simulink model "Simple_Model_Packaging_7_1"  (R2022b)
settings: Solver=VariableStepAuto  StartTime=0.0  StopTime=0.01  RelTol=1e-3
InitFcn:
  | Parameter_Initialize_7
undefined symbols (not defined in the file or in its folder): gcbh, magnitude, model, rcfiltgaincompat
libraries: simulink x2, commdigbbndfm2 x1, commdigbbndam3 x1, commfilt2 x1
settings Model: Creator=89778  LastModifiedBy=z0y

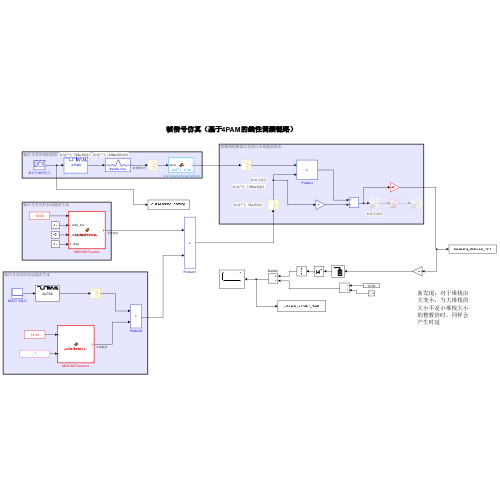
[thumbnail: Simulink's stored preview of the top-level diagram]
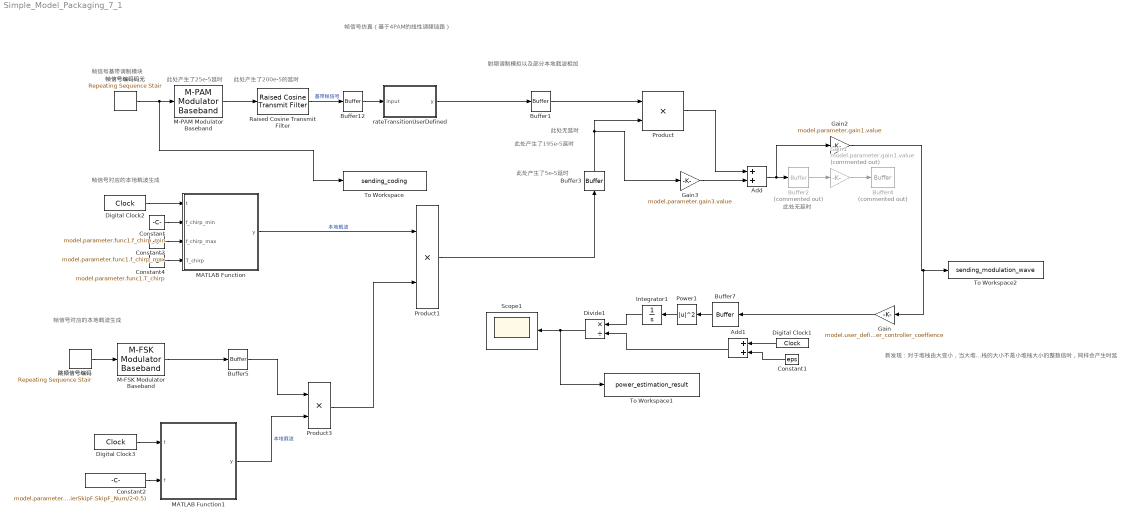
== system Simple_Model_Packaging_7_1 ==
  note: 帧信号仿真（基于4PAM的线性调频链路）
  note: 新发现：对于堆栈由大变小，当大堆栈的大小不是小堆栈大小的整数倍时，同样会产生时延
  note: 此处无延时
  note: 此处产生了25e-5延时
  note: 帧信号基带调制模块
  note: 此处产生了200e-5的延时
  note: 帧信号对应的本地载波生成
  note: 此处产生了195e-5延时
  note: 射频调制模拟以及部分本地载波相加
  note: 此处产生了5e-5延时
  note: 此处无延时
  note: 帧信号对应的本地载波生成
  Add : Sum
  Add1 : Sum
  Buffer1 : Buffer  N=model.parameter.Buffer1.Output_buffer_size  OutputFrames=off
  Buffer12 : Buffer  N=model.parameter.Buffer12.Output_buffer_size  OutputFrames=off
  Buffer2 : Buffer  Commented=on  N=model.parameter.Buffer2.Output_buffer_size  OutputFrames=off
  Buffer3 : Buffer  N=model.parameter.Buffer3.Output_buffer_size  OutputFrames=off
  Buffer4 : Buffer  Commented=on  N=model.parameter.Buffer4.Output_buffer_size  OutputFrames=off
  Buffer5 : Buffer  N=1  OutputFrames=off
  Buffer7 : Buffer  N=1  OutputFrames=off
  Constant : Constant  Value=model.parameter.func1.f_chirp_min
  Constant1 : Constant  Value=eps  SampleTime=model.parameter.channel_estimate_fs
  Constant2 : Constant  Value=model.parameter.CarrierSkipF.SkipF_distance*(model.parameter.CarrierSkipF.SkipF_Num/2-0.5)
  Constant3 : Constant  Value=model.parameter.func1.f_chirp_max
  Constant4 : Constant  Value=model.parameter.func1.T_chirp
  Digital Clock1 : DigitalClock  SampleTime=model.parameter.channel_estimate_fs
  Digital Clock2 : DigitalClock  SampleTime=model.parameter.Digital_Clock2.CarrierTs
  Digital Clock3 : DigitalClock  SampleTime=model.parameter.Digital_Clock2.CarrierTs
  Divide1 : Product  Inputs=*/
  Gain : Gain  Gain=model.user_defined.TR.Sig_power_controller_coeffience
  Gain1 : Gain  Commented=on  Gain=model.parameter.gain1.value
  Gain2 : Gain  Gain=model.parameter.gain1.value
  Gain3 : Gain  Gain=model.parameter.gain3.value
  Integrator1 : Integrator
  M-FSK Modulator Baseband : commdigbbndfm2/M-FSK Modulator Baseband  M=model.parameter.CarrierSkipF.SkipF_Num  InType=Integer  Enc=Binary  freqSep=model.parameter.CarrierSkipF.SkipF_distance  phaseType=Continuous  numSamp=ceil(model.parameter.CarrierSkipF.SkipF_time/model.parameter.Repeating_Sequence_Stair.CodeTs)*model.parameter.Raised_Cosine_Transmit_Filter.Output_samples_per_symbol  RateOptions=Enforce single-rate processing  outDataType=double
  M-PAM Modulator Baseband : commdigbbndam3/M-PAM Modulator Baseband  M=model.parameter.M_PAM_Modulator_Baseband.M_ary_number  InType=Integer  Enc=Gray  PowType=Min. distance between symbols  MinDist=model.parameter.M_PAM_Modulator_Baseband.Minimum_distance  AvgPow=1  PeakPow=1  outDtype=double  outWordLen=16  outUDDataType=sfix(16)  outFracLenMode=Best precision  outFracLen=15  outDataTypeStr=double  outLastDataTypeStr=double
  MATLAB Function : MATLAB Function  InitFcn=|  TreatAsAtomicUnit=on
      | f_chirp_min=4.8e6;
      | f_chirp_max=5.2e6;
      | T_chirp=4e-4;
  MATLAB Function1 : MATLAB Function  InitFcn=|  TreatAsAtomicUnit=on
      | f_chirp_min=4.8e6;
      | f_chirp_max=5.2e6;
      | T_chirp=4e-4;
  Power1 : Math  Operator=magnitude^2
  Product : Product
  Product1 : Product
  Product3 : Product
  Raised Cosine Transmit Filter : commfilt2/Raised Cosine Transmit Filter  filtType=Square root  R=model.parameter.Raised_Cosine_Transmit_Filter.Rolloff_factor  filtSpan=model.parameter.Raised_Cosine_Transmit_Filter.Filter_span_in_symbols  N=model.parameter.Raised_Cosine_Transmit_Filter.Output_samples_per_symbol  filterGain=rcfiltgaincompat(gcbh)  InputProcessing=Columns as channels (frame based)  RateOptions=Enforce single-rate processing  framing=Mute  checkCoeff=off  variableName=rcTxFilt  checkGain=Normalized  sampMode=Mute  saveAsFlag=0  currentFiltSpan=10  D=(10)/2  launchFVT=on  roundingMode=Floor  overflowMode=off  coeffDataTypeStr=Inherit: Same word length as input  coeffMin=[]  coeffMax=[]  coeffLastDataTypeStr=Inherit: Same word length as input  outputDataTypeStr=Inherit: Same as accumulator  outputMin=[]  outputMax=[]  outputLastDataTypeStr=Inherit: Same as accumulator
  Scope1 : Scope
  To Workspace : ToWorkspace  VariableName=sending_coding  SaveFormat=Timeseries  SampleTime=-1
  To Workspace1 : ToWorkspace  VariableName=power_estimation_result  SaveFormat=Timeseries  SampleTime=-1
  To Workspace2 : ToWorkspace  VariableName=sending_modulation_wave  SaveFormat=Timeseries  SampleTime=-1
  rateTransitionUserDefined : MATLAB Function  TreatAsAtomicUnit=on
  帧信号编码码元 : simulink/Sources/Repeating Sequence Stair  OutValues=model.parameter.Repeating_Sequence_Stair.output_vector  tsamp=model.parameter.Repeating_Sequence_Stair.CodeTs  OutMin=[]  OutMax=[]  OutDataTypeStr=double  OutputDataTypeScalingMode=double  OutDataType=fixdt(0,8)  ConRadixGroup=Best Precision: Vector-wise  OutScaling=2^-12
  跳频信号编码 : simulink/Sources/Repeating Sequence Stair  OutValues=model.parameter.CarrierSkipF.SkipF_vector  tsamp=model.parameter.Digital_Clock2.CarrierTs*ceil(model.parameter.CarrierSkipF.SkipF_time/model.parameter.Repeating_Sequence_Stair.CodeTs)*model.parameter.Raised_Cosine_Transmit_Filter.Output_samples_per_symbol  OutMin=[]  OutMax=[]  OutDataTypeStr=double  OutputDataTypeScalingMode=double  OutDataType=fixdt(0,8)  ConRadixGroup=Best Precision: Vector-wise  OutScaling=2^-12
  wires:
  Add1/1 -> Divide1/2
  Constant1/1 -> Add1/2
  Digital Clock1/1 -> Add1/1
  Power1/1 -> Integrator1/1
  Integrator1/1 -> Divide1/1
  Divide1/1 -> To Workspace1/1, Scope1/1
  Buffer7/1 -> Power1/1
  Buffer2/1 -> Gain1/1
  Buffer12/1 -> rateTransitionUserDefined/1(input)
  rateTransitionUserDefined/1(y) -> Buffer1/1
  Raised Cosine Transmit Filter/1 -> Buffer12/1  "基带帧信号"
  M-PAM Modulator Baseband/1 -> Raised Cosine Transmit Filter/1
  Digital Clock2/1 -> MATLAB Function/1(t)
  Buffer1/1 -> Product/1
  Add/1 -> Gain2/1, Buffer2/1
  Gain3/1 -> Add/2
  Product/1 -> Add/1
  Gain1/1 -> Buffer4/1
  Buffer3/1 -> Product/2, Gain3/1
  帧信号编码码元/1 -> To Workspace/1, M-PAM Modulator Baseband/1
  Constant/1 -> MATLAB Function/2(f_chirp_min)
  Constant3/1 -> MATLAB Function/3(f_chirp_max)
  Constant4/1 -> MATLAB Function/4(T_chirp)
  Gain/1 -> Buffer7/1
  Gain2/1 -> Gain/1, To Workspace2/1
  MATLAB Function/1(y) -> Product1/1  "本地载波"
  Product1/1 -> Buffer3/1
  M-FSK Modulator Baseband/1 -> Buffer5/1
  Constant2/1 -> MATLAB Function1/2(f)
  Digital Clock3/1 -> MATLAB Function1/1(t)
  MATLAB Function1/1(y) -> Product3/2  "本地载波"
  跳频信号编码/1 -> M-FSK Modulator Baseband/1
  Buffer5/1 -> Product3/1
  Product3/1 -> Product1/2

== matlab function Simple_Model_Packaging_7_1/MATLAB Function ==
  data: y output; t input; f_chirp_min input; f_chirp_max input; T_chirp input
% function y = carrierGenerator(t)
%     fc = 5e6;
%     y = exp(1i*2*pi*fc*t);

function y = carrierGenerator(t, f_chirp_min, f_chirp_max, T_chirp)
    k_chirp = (f_chirp_max-f_chirp_min)/T_chirp;
    t = mod(t,T_chirp);
    y = exp(1i*2*pi*(f_chirp_min*t+0.5*k_chirp*t^2));

end

== matlab function Simple_Model_Packaging_7_1/rateTransitionUserDefined ==
  data: y output; input input
% function y = carrierGenerator(t)
%     fc = 5e6;
%     y = exp(1i*2*pi*fc*t);

function y = rateTransition(input)
    p = 1;
    q = 1;
    y = resample(input,p,q);
%     y(1:100) = repmat(y(100),1,100);
%     y(end-99:end) = repmat(y(end-99),1,100);
end

== matlab function Simple_Model_Packaging_7_1/MATLAB Function1 ==
  data: y output; t input; f input
% function y = carrierGenerator(t)
%     fc = 5e6;
%     y = exp(1i*2*pi*fc*t);

function y = carrierGenerator(t, f)
    y = exp(1i*2*pi*f*t);
end
